simulink model "relative_distance_tracking3"  (R2018b)
settings: Solver=FixedStepAuto  StartTime=0.0  StopTime=40  FixedStep=dt  RelTol=1e-3
values from neighbouring files (symbols this model uses):
  C = [0 1]    [relative_distance_design2.m]
  CA = C*A    [relative_distance_design2.m]
  d0_ego = 0    [relative_distance_design2.m]
  d0_other = d0_ego + del_d0    (= 60)    [relative_distance_design2.m]
  del_d0 = 60    [relative_distance_design2.m]
  fc = 0.5    [relative_distance_design2.m]
  fps2mph = 1/mph2fps    (= 0.680272108844)    [relative_distance_design2.m]
  g = 32.2    [relative_distance_design2.m]
  invCB = inv(C*B)    [relative_distance_design2.m]
  Ka = 8    [relative_distance_design2.m]
  Kd = 2    [relative_distance_design2.m]
  Kv = 4    [relative_distance_design2.m]
  max_accel = 0.6*g    (= 19.32)    [relative_distance_design2.m]
  min_accel = -0.6*g    (= -19.32)    [relative_distance_design2.m]
  mph2fps = 1.47    [relative_distance_design2.m]
  v0_ego = 0*mph2fps    (= 0)    [relative_distance_design2.m]
  v0_other = v0_ego    (= 0)    [relative_distance_design2.m]
  v_other = v0_other + del_v0    (= 14.7)    [relative_distance_design2.m]
settings Model: Creator=suvo.ganguli  LastModifiedBy=suvo.ganguli

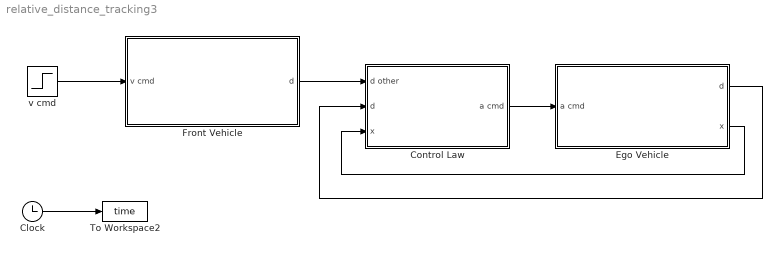
== system relative_distance_tracking3 ==
  Clock : Clock
  Control Law : Subsystem
  Ego Vehicle : Subsystem
  Front Vehicle : Subsystem
  To Workspace2 : ToWorkspace  VariableName=time  SampleTime=-1
  "v cmd " : Step  Before=v0_other  After=v_other  SampleTime=0
  wires:
  Clock/1 -> To Workspace2/1
  Control Law/1(a cmd) -> Ego Vehicle/1(a cmd)
  Ego Vehicle/2(x) -> Control Law/3(x)
  "v cmd "/1 -> Front Vehicle/1(v cmd)
  Ego Vehicle/1(d) -> Control Law/2(d)
  Front Vehicle/1(d) -> Control Law/1(d other)

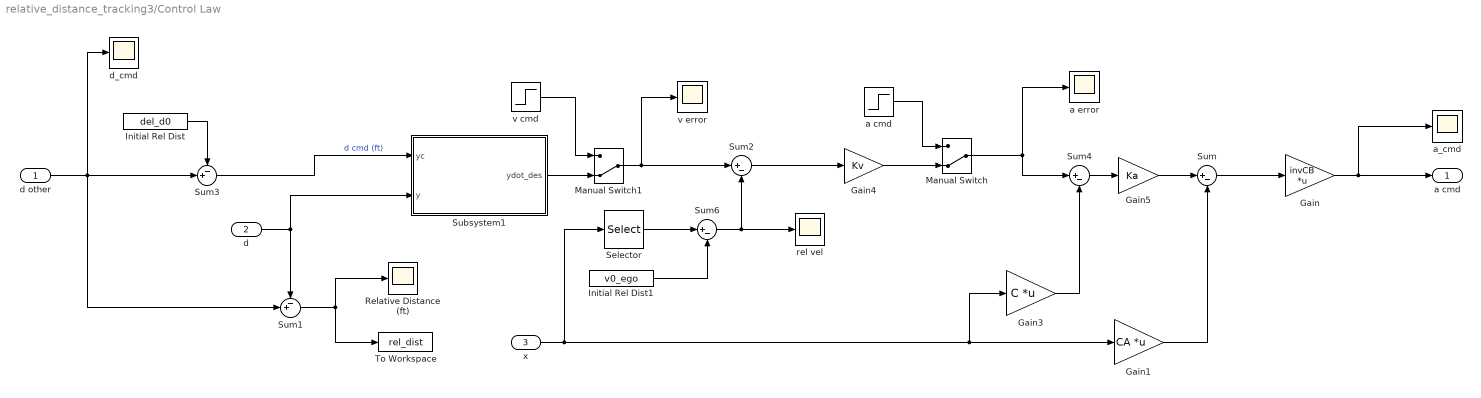
== system relative_distance_tracking3/Control Law ==
  d other : Inport
  d : Inport  Port=2
  x : Inport  Port=3
  Gain : Gain  Gain=invCB  Multiplication=Matrix(K*u)
  Gain1 : Gain  Gain=CA  Multiplication=Matrix(K*u)
  Gain3 : Gain  Gain=C  Multiplication=Matrix(K*u)
  Gain4 : Gain  Gain=Kv
  Gain5 : Gain  Gain=Ka
  Initial Rel Dist : Constant  Value=del_d0
  Initial Rel Dist1 : Constant  Value=v0_ego
  Manual Switch : ManualSwitch  CurrentSetting=0
  Manual Switch1 : ManualSwitch  CurrentSetting=0
  Relative Distance (ft) : Scope
  Selector : Selector  InputPortWidth=2  IndexOptions=Index vector (dialog)  Indices=1  OutputSizes=1
  Subsystem1 : Subsystem
  Sum{,2,4,6} (4 alike) : Sum  Inputs=|+-
  Sum1 : Sum  Inputs=-+|
  Sum3 : Sum  Inputs=-+|
  To Workspace : ToWorkspace  VariableName=rel_dist  SaveFormat=Timeseries  SampleTime=-1
  "a cmd " : Step  SampleTime=0
  a error : Scope
  a_cmd : Scope
  d_cmd : Scope
  rel vel : Scope
  v cmd : Step  Before=v0_ego  After=v0_ego + 10*mph2fps  SampleTime=0
  v error : Scope
  a cmd : Outport
  wires:
  x/1 -> Selector/1, Gain3/1, Gain1/1
  Gain5/1 -> Sum/1
  Gain1/1 -> Sum/2
  Gain/1 -> a cmd/1, a_cmd/1
  d other/1 -> Sum1/2, Sum3/2, d_cmd/1
  Manual Switch/1 -> Sum4/1, a error/1
  "a cmd "/1 -> Manual Switch/1
  Sum/1 -> Gain/1
  Gain4/1 -> Manual Switch/2
  Sum2/1 -> Gain4/1
  Manual Switch1/1 -> v error/1, Sum2/1
  v cmd/1 -> Manual Switch1/1
  Initial Rel Dist/1 -> Sum3/1
  Gain3/1 -> Sum4/2
  Sum4/1 -> Gain5/1
  Subsystem1/1(ydot_des) -> Manual Switch1/2
  Sum3/1 -> Subsystem1/1(yc)  "d cmd (ft)"
  d/1 -> Sum1/1, Subsystem1/2(y)
  Sum1/1 -> Relative Distance (ft)/1, To Workspace/1
  Sum6/1 -> Sum2/2, rel vel/1
  Selector/1 -> Sum6/1
  Initial Rel Dist1/1 -> Sum6/2

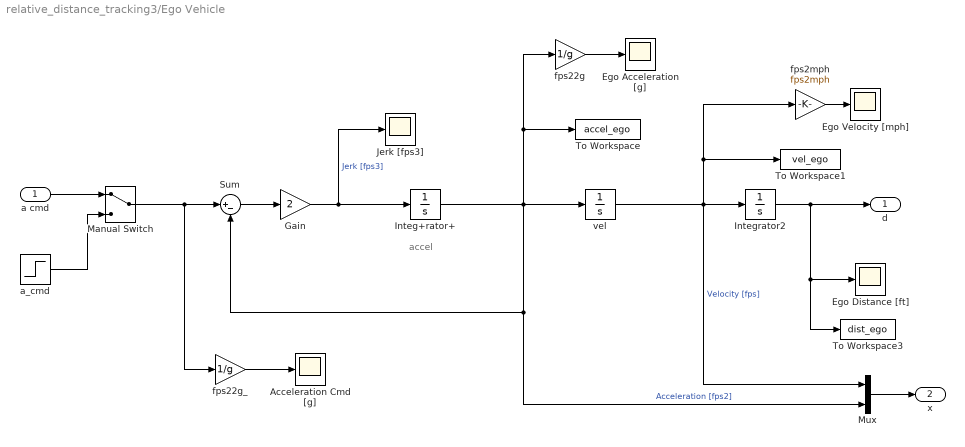
== system relative_distance_tracking3/Ego Vehicle ==
  note: accel
  a cmd : Inport
  Acceleration Cmd [g] : Scope
  Ego Acceleration [g] : Scope
  Ego Distance [ft] : Scope
  Ego Velocity [mph] : Scope
  Gain : Gain  Gain=2
  Integ+rator+ : Integrator  LimitOutput=on  UpperSaturationLimit=max_accel  LowerSaturationLimit=min_accel
  Integrator2 : Integrator  InitialCondition=d0_ego
  Jerk [fps3] : Scope
  Manual Switch : ManualSwitch
  Mux : Mux  Inputs=2
  Sum : Sum  Inputs=|+-
  To Workspace : ToWorkspace  VariableName=accel_ego  SampleTime=-1
  To Workspace1 : ToWorkspace  VariableName=vel_ego  SampleTime=-1
  To Workspace3 : ToWorkspace  VariableName=dist_ego  SampleTime=-1
  a_cmd : Step  SampleTime=0
  fps22g : Gain  Gain=1/g
  fps22g_ : Gain  Gain=1/g
  fps2mph : Gain  Gain=fps2mph
  vel : Integrator  InitialCondition=v0_ego
  d : Outport
  x : Outport  Port=2
  wires:
  Gain/1 -> Jerk [fps3]/1, Integ+rator+/1  "Jerk [fps3]"
  fps2mph/1 -> Ego Velocity [mph]/1
  vel/1 -> Mux/1, Integrator2/1, To Workspace1/1, fps2mph/1  "Velocity [fps]"
  Sum/1 -> Gain/1
  Integ+rator+/1 -> vel/1, To Workspace/1, fps22g/1, Mux/2, Sum/2  "Acceleration [fps2]"
  Integrator2/1 -> Ego Distance [ft]/1, To Workspace3/1, d/1
  fps22g/1 -> Ego Acceleration [g]/1
  Manual Switch/1 -> fps22g_/1, Sum/1
  a_cmd/1 -> Manual Switch/2
  a cmd/1 -> Manual Switch/1
  Mux/1 -> x/1
  fps22g_/1 -> Acceleration Cmd [g]/1

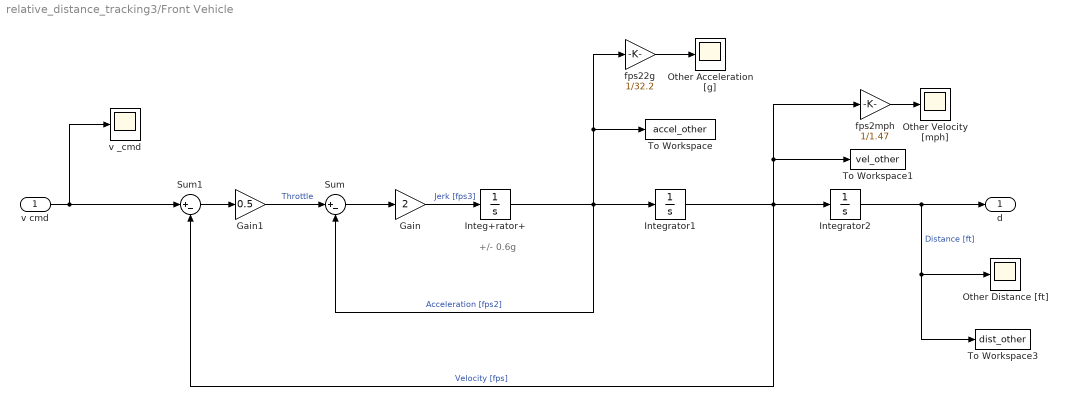
== system relative_distance_tracking3/Front Vehicle ==
  note: +/- 0.6g
  v cmd : Inport
  Gain : Gain  Gain=2
  Gain1 : Gain  Gain=0.5
  Integ+rator+ : Integrator  LimitOutput=on  UpperSaturationLimit=max_accel  LowerSaturationLimit=min_accel
  Integrator1 : Integrator  InitialCondition=v0_other
  Integrator2 : Integrator  InitialCondition=d0_other
  Other Acceleration [g] : Scope
  Other Distance [ft] : Scope
  Other Velocity [mph] : Scope
  Sum : Sum  Inputs=|+-
  Sum1 : Sum  Inputs=|+-
  To Workspace : ToWorkspace  VariableName=accel_other  SampleTime=-1
  To Workspace1 : ToWorkspace  VariableName=vel_other  SampleTime=-1
  To Workspace3 : ToWorkspace  VariableName=dist_other  SampleTime=-1
  fps22g : Gain  Gain=1/32.2
  fps2mph : Gain  Gain=1/1.47
  v _cmd : Scope
  d : Outport
  wires:
  Gain1/1 -> Sum/1  "Throttle"
  v cmd/1 -> Sum1/1, v _cmd/1
  fps22g/1 -> Other Acceleration [g]/1
  Sum1/1 -> Gain1/1
  Integ+rator+/1 -> Sum/2, fps22g/1, To Workspace/1, Integrator1/1  "Acceleration [fps2]"
  Sum/1 -> Gain/1
  Integrator1/1 -> fps2mph/1, To Workspace1/1, Integrator2/1, Sum1/2  "Velocity [fps]"
  fps2mph/1 -> Other Velocity [mph]/1
  Gain/1 -> Integ+rator+/1  "Jerk [fps3]"
  Integrator2/1 -> d/1, To Workspace3/1, Other Distance [ft]/1  "Distance [ft]"

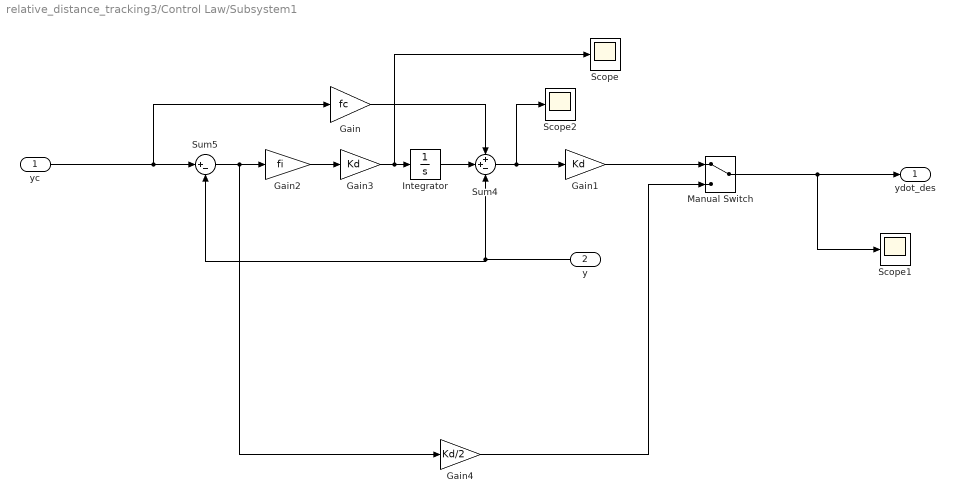
== system relative_distance_tracking3/Control Law/Subsystem1 ==
  yc : Inport
  y : Inport  Port=2
  Gain : Gain  Gain=fc
  Gain1 : Gain  Gain=Kd
  Gain2 : Gain  Gain=fi
  Gain3 : Gain  Gain=Kd
  Gain4 : Gain  Gain=Kd/2
  Integrator : Integrator
  Manual Switch : ManualSwitch
  Scope : Scope
  Scope1 : Scope
  Scope2 : Scope
  Sum4 : Sum  Inputs=++-
  Sum5 : Sum  Inputs=|+-
  ydot_des : Outport
  wires:
  Sum4/1 -> Scope2/1, Gain1/1
  Gain2/1 -> Gain3/1
  Sum5/1 -> Gain4/1, Gain2/1
  yc/1 -> Gain/1, Sum5/1
  Integrator/1 -> Sum4/2
  Gain/1 -> Sum4/1
  y/1 -> Sum5/2, Sum4/3
  Gain3/1 -> Scope/1, Integrator/1
  Gain1/1 -> Manual Switch/1
  Manual Switch/1 -> Scope1/1, ydot_des/1
  Gain4/1 -> Manual Switch/2
